simulink model "DAB_SIMULINK"  (R2024b)
settings: Solver=ode23s  StartTime=0.0  StopTime=0.0001  MaxStep=1e-4  RelTol=1e-3
libraries: spsIGBTDiodeLib x8, spsVoltageMeasurementLib x4, spsSeriesRLCBranchLib x3, spsCurrentMeasurementLib x1, spsDCVoltageSourceLib x1, spsLinearTransformerLib x1, spspowerguiLib x1
settings Model: Creator=Le'novo  LastModifiedBy=wei13
settings SolverCC: AlgebraicLoopSolver=TrustRegion
settings DataIOCC: ReturnWorkspaceOutputs=off
settings DebuggingCC: UnconnectedInputMsg=warning  UnconnectedOutputMsg=warning  UnconnectedLineMsg=warning  ArithmeticOperatorsInVariantConditions=warning
settings ModelReferenceCC: EnableRefExpFcnMdlSchedulingChecks=on
settings SFSimCC: SimUseLocalCustomCode=off  CustomCodeUndefinedFunction=UseInterfaceOnly
settings RTWCC: RTWUseLocalCustomCode=off  GPUComputeCapability=3.5
settings CodeAppCC: StateflowObjectComments=on
settings SimscapeCC: SimscapeNormalizeSystem=off

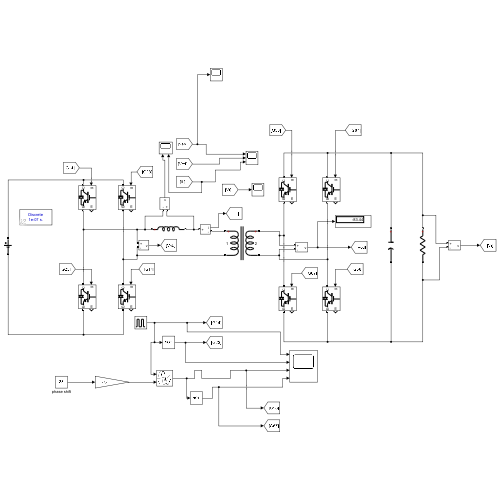
[thumbnail: Simulink's stored preview of the top-level diagram]
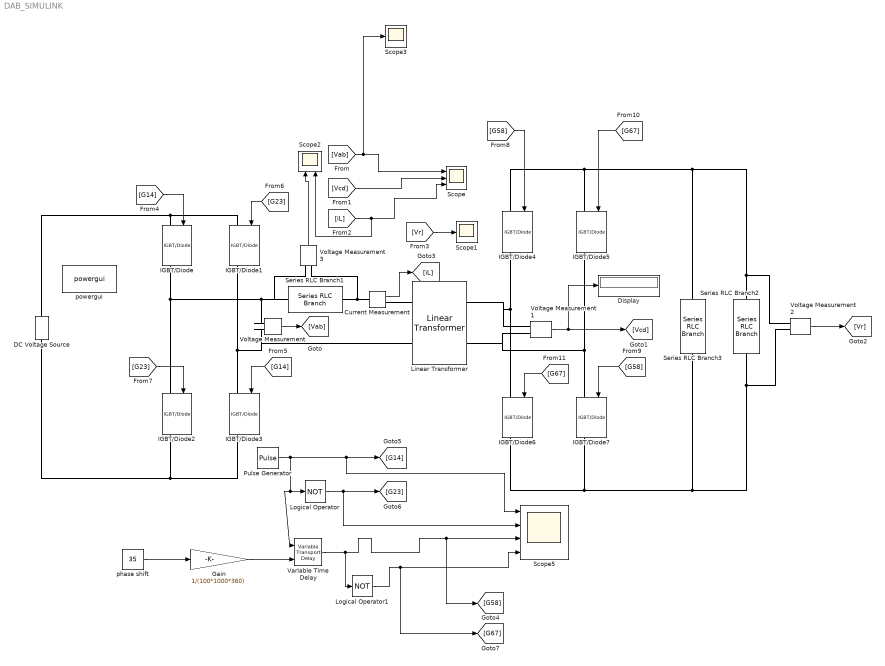
== system DAB_SIMULINK ==
  Current Measurement : spsCurrentMeasurementLib/Current Measurement  PhasorSimulation=off  OutputType=Complex  PSBequivalent=0
  DC Voltage Source : spsDCVoltageSourceLib/DC Voltage Source  Amplitude=48  Measurements=None
  Display : Display
  Gain : Gain  Gain=1/(100*1000*360)
  IGBT/Diode{,1..7} (8 alike) : spsIGBTDiodeLib/IGBT//Diode  Ron=1e-3  Rs=1e5  Cs=inf  Measurements=on
  Linear Transformer : spsLinearTransformerLib/Linear Transformer  UNITS=SI  NominalPower=[ 250e6 100*1000 ]  winding1=[100 1e-9 1e-9]  winding2=[300 1e-9 1e-9]  ThreeWindings=off  winding3=[3.15e+05 315.06 3.1922e-08]  RmLm=[1.0805e+07 2866]  Measurements=None  DataType=on
  Logical Operator : Logic  Operator=NOT  AllPortsSameDT=off  OutDataTypeStr=boolean
  Logical Operator1 : Logic  Operator=NOT  AllPortsSameDT=off  OutDataTypeStr=boolean
  Pulse Generator : DiscretePulseGenerator  PulseType=Time based  Period=1/(100*1000)  PulseWidth=50
  Scope : Scope  NumInputPorts=3
  Scope1 : Scope
  Scope2 : Scope  NumInputPorts=2
  Scope3 : Scope
  Scope5 : Scope  NumInputPorts=4
  Series RLC Branch1 : spsSeriesRLCBranchLib/Series RLC Branch  LConnTagsString=__new0  RConnTagsString=__new0  BranchType=L  Resistance=1  Inductance=10e-08  SetiL0=off  InitialCurrent=0  Capacitance=1e-6  Setx0=off  InitialVoltage=0  Measurements=None
  Series RLC Branch2 : spsSeriesRLCBranchLib/Series RLC Branch  LConnTagsString=__new0  RConnTagsString=__new0  BranchType=R  Resistance=1  Inductance=1e-3  SetiL0=off  InitialCurrent=0  Capacitance=1e-6  Setx0=off  InitialVoltage=0  Measurements=None
  Series RLC Branch3 : spsSeriesRLCBranchLib/Series RLC Branch  LConnTagsString=__new0  RConnTagsString=__new0  BranchType=C  Resistance=1  Inductance=1e-3  SetiL0=off  InitialCurrent=0  Capacitance=100e-6  Setx0=off  InitialVoltage=0  Measurements=None
  Variable Time Delay : VariableTransportDelay  MaximumDelay=10
  Voltage Measurement{,1..3} (4 alike) : spsVoltageMeasurementLib/Voltage Measurement  PhasorSimulation=off  OutputType=Complex  PSBequivalent=0
  "phase shift " : Constant  Value=35
  powergui : spspowerguiLib/powergui  Priority=1  SimulationMode=Discrete  SampleTime=1/100E3/100  frequency=60  Iterations=50  frequencyindice=0  Pbase=100e6  ErrMax=1e-4  UnitsV=kV  UnitsW=MW  buscounter=0  FunctionMessages=off  echomessages=off  EnableUseOfTLC=off  CurrentSourceSwitches=off  DisableSnubberDevices=off  DisableRonSwitches=off  DisableVfSwitches=off  DisplayEquations=off  AutomaticDiscreteSolvers=off  SolverType=Tustin/Backward Euler (TBE)  Interpol=off  ExternalGateDelay=off  methode=off  Ts=100  x0status=blocks  SPID=on  SwTol=0  HookPort=off  NonlinearTolerance=1e-4  nMaxIteration=100  ContinueOnMaxIteration=off  RestoreLinks=warning  ResistiveCurrentMeasurement=off  Frange=[0:2:500]  Ylog=off  Xlog=on  ShowGrid=off  save=off  variable=ZData  structure=0  ZoomFFT=off  StartTime=0.0  cycles=1  DisplayStyle=1  fundamental=60  FreqAxis=off  MaxFrequency=1000  frequencyindicesteady=1  RmsSteady=1  display=off
  wires:
  Voltage Measurement/1 -> [Vab]
  Current Measurement/1 -> [iL]
  Voltage Measurement1/1 -> Display/1, [Vcd]
  Voltage Measurement2/1 -> [Vr]
  [Vr] -> Scope1/1
  [Vab] -> Scope3/1, Scope/1
  [Vcd] -> Scope/2
  [iL] -> Scope2/2, Scope/3
  [G14] -> IGBT/Diode/1
  [G23] -> IGBT/Diode1/1
  [G14] -> IGBT/Diode3/1
  [G23] -> IGBT/Diode2/1
  Pulse Generator/1 -> Variable Time Delay/1, Logical Operator/1, Scope5/1, [G14]
  Logical Operator/1 -> Scope5/2, [G23]
  "phase shift "/1 -> Gain/1
  Logical Operator1/1 -> [G67], Scope5/4
  Gain/1 -> Variable Time Delay/2
  Variable Time Delay/1 -> Logical Operator1/1, [G58], Scope5/3
  [G58] -> IGBT/Diode4/1
  [G67] -> IGBT/Diode5/1
  [G58] -> IGBT/Diode7/1
  [G67] -> IGBT/Diode6/1
  Voltage Measurement3/1 -> Scope2/1
  connections:
  IGBT/Diode/RConn1 -- Voltage Measurement3/LConn2 -- Series RLC Branch1/LConn1 -- Voltage Measurement/LConn1 -- IGBT/Diode2/LConn1
  IGBT/Diode1/RConn1 -- Voltage Measurement/LConn2 -- Linear Transformer/LConn2 -- IGBT/Diode3/LConn1
  DC Voltage Source/RConn1 -- IGBT/Diode1/LConn1 -- IGBT/Diode/LConn1
  DC Voltage Source/LConn1 -- IGBT/Diode2/RConn1 -- IGBT/Diode3/RConn1
  Series RLC Branch1/RConn1 -- Voltage Measurement3/LConn1 -- Current Measurement/LConn1
  Linear Transformer/LConn1 -- Current Measurement/RConn1
  IGBT/Diode4/RConn1 -- Voltage Measurement1/LConn1 -- Linear Transformer/RConn1 -- IGBT/Diode6/LConn1
  IGBT/Diode5/RConn1 -- Voltage Measurement1/LConn2 -- Linear Transformer/RConn2 -- IGBT/Diode7/LConn1
  IGBT/Diode5/LConn1 -- IGBT/Diode4/LConn1 -- Series RLC Branch3/LConn1 -- Voltage Measurement2/LConn1 -- Series RLC Branch2/LConn1
  IGBT/Diode6/RConn1 -- IGBT/Diode7/RConn1 -- Series RLC Branch3/RConn1 -- Voltage Measurement2/LConn2 -- Series RLC Branch2/RConn1
